simulink subsystem "FTC_UnknownV3"  (R2022a)
settings: Solver=VariableStepAuto  StartTime=0.0  StopTime=10.0  RelTol=1e-3
values from neighbouring files (symbols this model uses):
  g = (9.8)    (= 9.8)    [H250_LOEKnown_400HzParam.m]    (also in H250_LOEUnknown_400HzParam.m; H333_LOEKnown_400HzParam.m)
  J = (diag([0.0056 0.0056 0.0104]))    [H250_LOEKnown_400HzParam.m]    (also in H250_LOEUnknown_400HzParam.m; H333_LOEKnown_400HzParam.m = (diag([0.012 0.0120 0.02])))
  M = ([ 1          1          1         1 ... (first row only)    [H250_LOEKnown_400HzParam.m]    (also in H250_LOEUnknown_400HzParam.m; H333_LOEKnown_400HzParam.m)
  m = (0.752)    (= 0.752)    [H250_LOEKnown_400HzParam.m]    (also in H250_LOEUnknown_400HzParam.m; H333_LOEKnown_400HzParam.m = 1.13)
  MY_ATT_P = Pixhawk_CSC.Parameter( {single(8), 'MY_ATT_P'}  )    [H250_LOEKnown_400HzParam.m]    (also in H250_LOEUnknown_400HzParam.m = Pixhawk_CSC.Parameter( {single(3), 'MY_ATT_P'}  ); H333_LOEKnown_400HzParam.m)
  MY_ATT_P_YAW = Pixhawk_CSC.Parameter( {single(0), 'MY_ATT_P_YAW'}  )    [H250_LOEKnown_400HzParam.m]    (also in H250_LOEUnknown_400HzParam.m = Pixhawk_CSC.Parameter( {single(0.0), 'MY_ATT_P_YAW'}  ); H333_LOEKnown_400HzParam.m)
  MY_K_CP = Pixhawk_CSC.Parameter({single(0.7), 'MY_K_CP'} )    [H250_LOEUnknown_400HzParam.m]
  MY_POS_P = Pixhawk_CSC.Parameter( {single(0.5), 'MY_POS_P'}  )    [H250_LOEKnown_400HzParam.m]    (also in H250_LOEUnknown_400HzParam.m; H333_LOEKnown_400HzParam.m)
  MY_RATE_P = Pixhawk_CSC.Parameter( {single(12), 'MY_RATE_P'}  )    [H250_LOEKnown_400HzParam.m]    (also in H250_LOEUnknown_400HzParam.m = Pixhawk_CSC.Parameter( {single(14), 'MY_RATE_P'}  ); H333_LOEKnown_400HzParam.m)
  MY_RATE_P_YAW = Pixhawk_CSC.Parameter( {single(0.3), 'MY_RATE_P_YAW'}  )    [H250_LOEKnown_400HzParam.m]    (also in H250_LOEUnknown_400HzParam.m = Pixhawk_CSC.Parameter( {single(0.0), 'MY_RATE_P_YAW'}  ); H333_LOEKnown_400HzParam.m)
  MY_SAT_AD = Pixhawk_CSC.Parameter({single(0.13), 'MY_SAT_AD'} )    [H250_LOEKnown_400HzParam.m]    (also in H250_LOEUnknown_400HzParam.m; H333_LOEKnown_400HzParam.m)
  MY_TAU_P_A = Pixhawk_CSC.Parameter( {single(0), 'MY_TAU_P_A'}  )    [H250_LOEKnown_400HzParam.m]    (also in H250_LOEUnknown_400HzParam.m = Pixhawk_CSC.Parameter( {single(0.0), 'MY_TAU_P_A'}  ); H333_LOEKnown_400HzParam.m)
  MY_TAU_P_A_YAW = Pixhawk_CSC.Parameter( {single(0), 'MY_TAU_P_A_YAW'}  )    [H250_LOEKnown_400HzParam.m]    (also in H250_LOEUnknown_400HzParam.m; H333_LOEKnown_400HzParam.m)
  MY_TAU_P_P = Pixhawk_CSC.Parameter( {single(1.5), 'MY_TAU_P_P'}  )    [H250_LOEKnown_400HzParam.m]    (also in H250_LOEUnknown_400HzParam.m = Pixhawk_CSC.Parameter( {single(1.3), 'MY_TAU_P_P'}  ); H333_LOEKnown_400HzParam.m)
  MY_TAU_P_P_YAW = Pixhawk_CSC.Parameter( {single(0.1), 'MY_TAU_P_P_YAW'}  )    [H250_LOEKnown_400HzParam.m]    (also in H250_LOEUnknown_400HzParam.m; H333_LOEKnown_400HzParam.m)
  MY_VEL_P = Pixhawk_CSC.Parameter( {single(0.8), 'MY_VEL_P'}  )    [H250_LOEKnown_400HzParam.m]    (also in H250_LOEUnknown_400HzParam.m; H333_LOEKnown_400HzParam.m)
  T00 = single([m*g/4 m*g/4 m*g/4 m*g/4]')    [H250_LOEKnown_400HzParam.m]    (also in H250_LOEUnknown_400HzParam.m; H333_LOEKnown_400HzParam.m)
  Tf = 0.06    [H250_LOEKnown_400HzParam.m]    (also in H250_LOEUnknown_400HzParam.m; H333_LOEKnown_400HzParam.m)
  Tmotorbar = (0.035)    (= 0.035)    [H250_LOEKnown_400HzParam.m]    (also in H250_LOEUnknown_400HzParam.m = 0.032; H333_LOEKnown_400HzParam.m)
  Ts = 1/400    (= 0.0025)    [H250_LOEKnown_400HzParam.m]    (also in H250_LOEUnknown_400HzParam.m; H333_LOEKnown_400HzParam.m)
undefined symbols (not defined in the file or in its folder): MY_POS_ALT, MY_VEL_ALT
libraries: discretizing x13, slpidlib x4, simulink x2, pixhawk_slib_uORB_RW x1
(part 2 of 2)

== matlab function FTC_UnknownV3/innerloop/Att ==
  data: e input; w input; eulerangle input; pqrd output; ATT_P input; ATT_P_SCALE input
function pqrd  = fcn(e, w, eulerangle, ATT_P, ATT_P_SCALE)
%% 角度控制1
% h1 = n3(1);
% h2 = n3(2);
% h3 = n3(3);
% h1d = n3d(1);
% h2d = n3d(2);
% h3d = n3d(3);
% we = Reb*w;
% k1 = single(5);
% epqd = [0 -1/h3; 1/h3 0]*[k1*(h1d-h1)+h2*we(3);k1*(h2d-h2)-h1*we(3)];
% 
% psid = single(0);
% rd = k1*0.3*(psid - psi);
% 
% Rbe = Reb';
% erd = (rd - Rbe(3,1)*epqd(1) - Rbe(3,2)*epqd(2))/Rbe(3,3);
% 
% pqd = Rbe((1:2),:)*[epqd; erd];%计算出机体系下的pqd
% pqd = mysat(pqd,2);
% pqrd = [pqd;rd];
%% 角度控制2
e1 = e(1);
e2 = e(2);
% e1  = n3(1) - n3d(1);
% e2  = n3(2) - n3d(2); 
beta = atan2(e2,e1);
psi = eulerangle(1);
costheta = eulerangle(2);
cosphi = eulerangle(3);
k1 = ATT_P;
pqd = [ -k1*sqrt(e1^2+e2^2)*sin(psi-beta);%costheta
             -k1*sqrt(e1^2+e2^2)*cos(psi-beta)];%cosphi
pqd = mysatsingle(pqd,3);
psid = 0;
% rd = -k1*0.3*(psi-psid);
rd = -k1*ATT_P_SCALE*(psi-psid);
% rd = 0;
pqrd = [pqd;rd];

== matlab function FTC_UnknownV3/outerloop/Position2/MATLAB Function ==
  data: manualRC input; pos_d output; current_pos input; Ts input
function pos_d = fcn(manualRC, current_pos, Ts)
persistent desired_pos_static manualRC_last
if isempty(desired_pos_static)
    desired_pos_static = current_pos;
end
if isempty(manualRC_last)
    manualRC_last = single([0;0]);
end

if norm(manualRC)>0.01
    desired_pos_static = desired_pos_static + Ts*manualRC;
else
    if manualRC_last>0.01
        desired_pos_static = current_pos;
    end
end
manualRC_last = manualRC;
pos_d = desired_pos_static;

== matlab function FTC_UnknownV3/outerloop/d_z ==
  data: n3 input size=[3,1]; dvz input single size=1; T_ input single size=4; M input single size=[4,4]; m input single size=1; g input single size=1; dz output single size=1
function dz   = fcn(n3, dvz, T_, M, m, g)
dz  = m*(0.3*dvz-g)/n3(3)+M(1,:)*T_;

== matlab function FTC_UnknownV3/Subsystem2/MATLAB Function ==
  data: Reb input; eulerangle output
function eulerangle = fcn(Reb)
% 方位角计算
psi = atan2(Reb(2,1), Reb(1,1));
% 借助方位角快速计算出横滚俯仰角的余弦
costheta = Reb(1,1)/cos(psi);
cosphi = Reb(3,3)/costheta;
eulerangle = [psi; costheta; cosphi];

== matlab function FTC_UnknownV3/outerloop/Pos ==
  data: a_des_0 input single size=3; n3 input size=3; m input single size=1; fd output single size=1; g input single size=1; n3d output single size=[3,1]; ad output single size=3; SAT_AD input single size=1
function [fd, n3d, ad]  = fcn(a_des_0, n3, m, g, SAT_AD)
% 计算期望的主轴
    % a_des_g: 期望的电机产生总推力产生的加速度, 为了克服重力且重力方向是正方向所以推理克服重力应该是向上的,所以是-g 
    a_des_0_g = (a_des_0 - [single(0); single(0); g]);
    epsilon = max(  (sqrt(a_des_0_g(1)^2+a_des_0_g(2)^2)/abs(a_des_0_g(3)))/single(SAT_AD)  ,1);
    % 确保只压缩水平方向的加速度, 确保高度通道的加速的不会被饱和干扰, 做到真正的重力方向优先
    a_des_g = [1/epsilon 1/epsilon 1].*a_des_0_g';
    % 计算期望的主轴
    n3d = -(a_des_g')/norm(a_des_g);

    % 旧的方案
    % 计算饱和后的期望加速度
    ad = mysatsingle(a_des_0,single(SAT_AD)*g);
%     n3d = ([single(0); single(0); g]-ad)/norm([single(0); single(0); g]-ad);

% 计算期望的拉力
if n3d(3)==single(0)
    fd = single(0);
else
    % 旧方案
%     fd = m*(g-ad(3))/n3(3);
    % 新方案
    fd = m*(-a_des_g(3))/n3(3);

end
